simulink model "parcial_ej3_simu_20210906"  (R2021a)
settings: Solver=ode4  StartTime=0.0  StopTime=50  FixedStep=0.0001  RelTol=1e-3
libraries: cstblocks x2
settings Model: Creator=aghersin  LastModifiedBy=frand
settings SolverCC: AlgebraicLoopSolver=TrustRegion
settings DataIOCC: ReturnWorkspaceOutputs=off
settings OptimizationCC: LifeSpan=inf
settings DebuggingCC: SFExecutionAtInitializationDiag=none  SFMachineParentedDataDiag=warning  ArithmeticOperatorsInVariantConditions=warning
settings SFSimCC: SimUseLocalCustomCode=off  CustomCodeUndefinedFunction=UseInterfaceOnly
settings RTWCC: RTWUseLocalCustomCode=off
settings CodeAppCC: StateflowObjectComments=on

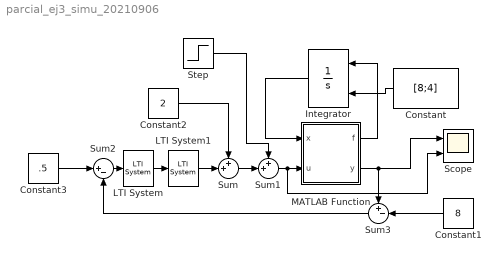
== system parcial_ej3_simu_20210906 ==
  Constant : Constant  Value=[8;4]
  Constant1 : Constant  Value=8
  Constant2 : Constant  Value=2
  Constant3 : Constant  Value=.5
  Integrator : Integrator  InitialConditionSource=external
  LTI System : cstblocks/LTI System  sys=C_simu  IC=[]
  LTI System1 : cstblocks/LTI System  sys=Pade  IC=[]
  MATLAB Function : MATLAB Function  TreatAsAtomicUnit=on
  Scope : Scope  NumInputPorts=2
  Step : Step  SampleTime=1
  Sum : Sum  Inputs=++|
  Sum1 : Sum  Inputs=++|
  Sum2 : Sum  Inputs=|+-
  Sum3 : Sum  Inputs=+-|
  wires:
  Integrator/1 -> MATLAB Function/1(x)
  MATLAB Function/1(f) -> Integrator/1
  Constant/1 -> Integrator/2
  MATLAB Function/2(y) -> Sum3/1, Scope/1
  Constant1/1 -> Sum3/2
  Constant2/1 -> Sum/1
  Sum2/1 -> LTI System/1
  Constant3/1 -> Sum2/1
  Sum3/1 -> Sum2/2
  LTI System/1 -> LTI System1/1
  LTI System1/1 -> Sum/2
  Sum/1 -> Sum1/2
  Sum1/1 -> Scope/2, MATLAB Function/2(u)
  Step/1 -> Sum1/1

== matlab function parcial_ej3_simu_20210906/MATLAB Function ==
  data: x input; u input; f output; y output
function [f,y] = fcn(x,u)

f1=u - sqrt(x(1)-x(2));
f2=sqrt(x(1)-x(2))-sqrt(x(2));
f=[f1;f2];

y=x(1);
